simulink model "E2_SimulacionNeumatico"  (R2022b)
settings: Solver=VariableStepAuto  StartTime=0.0  StopTime=10.0  MaxStep=0.0001  RelTol=1e-3
values from neighbouring files (symbols this model uses):
  b1 = 1000    [E2_Parametros.m]
  f = 0    [E2_Parametros.m]
  k1 = 16182    [E2_Parametros.m]
  k2 = 19000    [E2_Parametros.m]
  m1 = 290    [E2_Parametros.m]
  m2 = 59    [E2_Parametros.m]
settings Model: Creator=mluser  LastModifiedBy=mluser

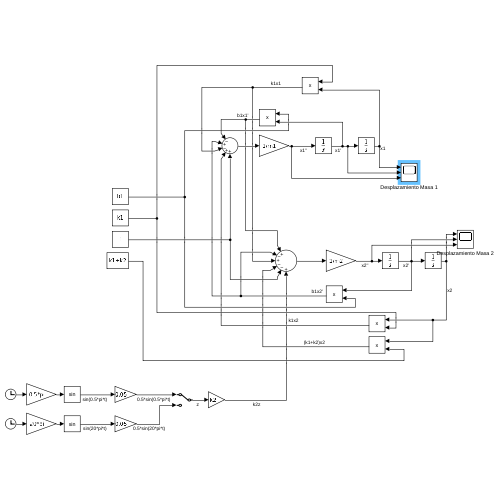
[thumbnail: Simulink's stored preview of the top-level diagram]
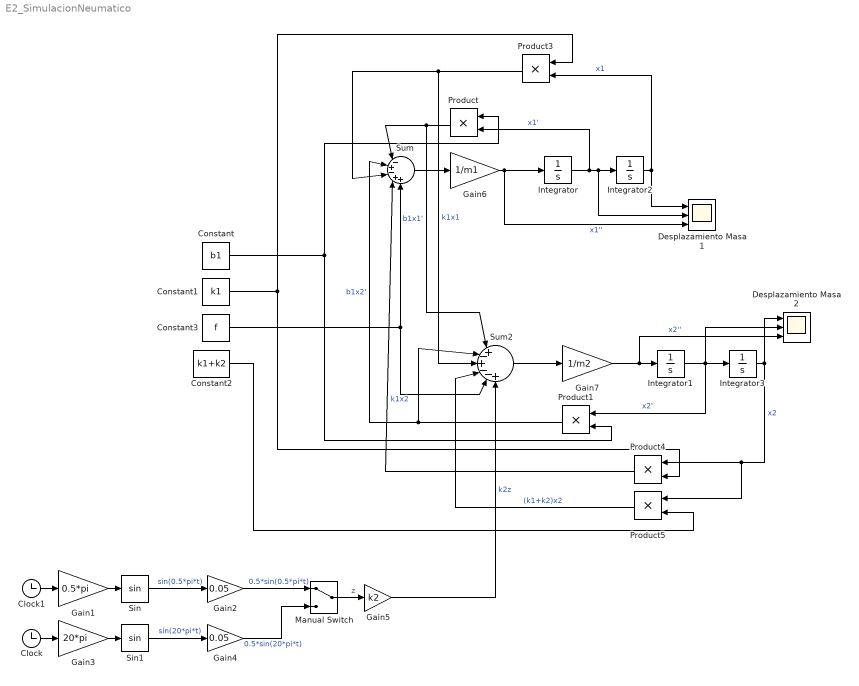
== system E2_SimulacionNeumatico ==
  Clock : Clock
  Clock1 : Clock
  Constant : Constant  Value=b1
  Constant1 : Constant  Value=k1
  Constant2 : Constant  Value=k1+k2
  Constant3 : Constant  Value=f
  Desplazamiento Masa 1 : Scope  NumInputPorts=3
  Desplazamiento Masa 2 : Scope  NumInputPorts=3
  Gain1 : Gain  Gain=0.5*pi
  Gain2 : Gain  Gain=0.05
  Gain3 : Gain  Gain=20*pi
  Gain4 : Gain  Gain=0.05
  Gain5 : Gain  Gain=k2
  Gain6 : Gain  Gain=1/m1
  Gain7 : Gain  Gain=1/m2
  Integrator{,1..3} (4 alike) : Integrator
  Manual Switch : ManualSwitch
  Product{,1,3..5} (5 alike) : Product
  Sin : Trigonometry
  Sin1 : Trigonometry
  Sum : Sum  Inputs=|-+-++
  Sum2 : Sum  Inputs=|+-+--+
  wires:
  Clock/1 -> Gain3/1
  Clock1/1 -> Gain1/1
  Gain1/1 -> Sin/1
  Sin/1 -> Gain2/1  "sin(0.5*pi*t)"
  Sin1/1 -> Gain4/1  "sin(20*pi*t)"
  Gain2/1 -> Manual Switch/1  "0.5*sin(0.5*pi*t)"
  Gain3/1 -> Sin1/1
  Gain4/1 -> Manual Switch/2  "0.5*sin(20*pi*t)"
  Manual Switch/1 -> Gain5/1  "z"
  Integrator1/1 -> Desplazamiento Masa 2/2, Product1/1, Integrator3/1  "x2'"
  Integrator2/1 -> Desplazamiento Masa 1/1, Product3/2  "x1"
  Integrator3/1 -> Desplazamiento Masa 2/1, Product5/1, Product4/1  "x2"
  Integrator/1 -> Product/2, Desplazamiento Masa 1/2, Integrator2/1  "x1'"
  Gain6/1 -> Desplazamiento Masa 1/3, Integrator/1  "x1''"
  Gain7/1 -> Desplazamiento Masa 2/3, Integrator1/1  "x2''"
  Sum/1 -> Gain6/1
  Sum2/1 -> Gain7/1
  Constant/1 -> Product1/2, Product/1
  Product/1 -> Sum2/1, Sum/1  "b1x1'"
  Product1/1 -> Sum2/2, Sum/2  "b1x2'"
  Constant1/1 -> Product4/2, Product3/1
  Product3/1 -> Sum/3, Sum2/3  "k1x1"
  Product4/1 -> Sum/4  "k1x2"
  Constant3/1 -> Sum/5, Sum2/5
  Gain5/1 -> Sum2/6  "k2z"
  Constant2/1 -> Product5/2
  Product5/1 -> Sum2/4  "(k1+k2)x2"
